simulink model "imageReceiveExample1"  (R2014a)
settings: Solver=FixedStepDiscrete  StartTime=0.0  StopTime=inf  RelTol=1e-3
undefined symbols (not defined in the file): gray, Rec, SDTV
libraries: dspmtrx3 x6, visionconversions x4, visionsinks x3, dspvision x2, ARdrone_video_lib x2
settings Model: xpc_rtwmakecfg_data=_jpeg_  Creator=Catarina  LastModifiedBy=Catarina

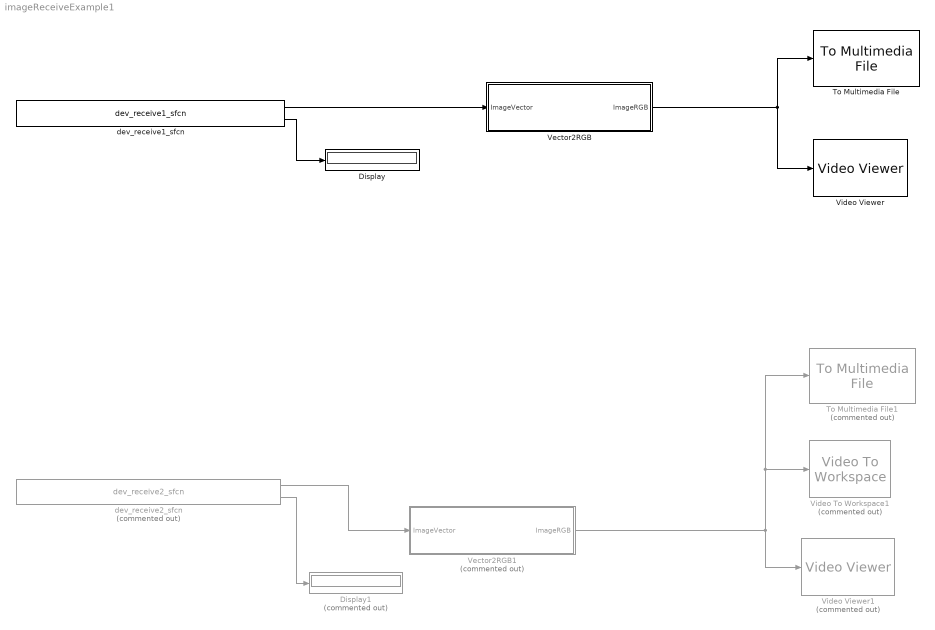
== system imageReceiveExample1 ==
  Display : Display
  Display1 : Display  Commented=on
  To Multimedia File : dspvision/To Multimedia File  outputFilename=output.avi  streamSelection=Video only  videoCompressor=None (uncompressed)  audioCompressor=None (uncompressed)  imagePorts=One multidimensional signal  fileType=AVI  audioDatatype=Determine from input data type  fourcc=RGB  videoQuality=75  mj2000CompFactor=10
  To Multimedia File1 : dspvision/To Multimedia File  Commented=on  outputFilename=output2.avi  streamSelection=Video only  videoCompressor=None (uncompressed)  audioCompressor=None (uncompressed)  imagePorts=One multidimensional signal  fileType=AVI  audioDatatype=Determine from input data type  fourcc=RGB  videoQuality=75  mj2000CompFactor=10
  Vector2RGB : Subsystem
  Vector2RGB1 : Subsystem  Commented=on
  Video To Workspace1 : visionsinks/Video To Workspace  Commented=on  VariableName=vout2  NumInputs=1  DataLimit=10  DecimationFactor=1  LogFi=off  InPortLabels=R|G|B
  Video Viewer : visionsinks/Video Viewer  inputType=Obsolete7b  imagePorts=One multidimensional signal  useColorMap=off  colormapValue=gray(256)  specRange=off  minInputVal=0  maxInputVal=255  FigPos=[1 1038 1920 938]  AxisZoom=on  trueSizedOnce=off  OpenAtMdlStart=on  DefaultConfigurationName=vipscopes.VideoViewerScopeCfg
  Video Viewer1 : visionsinks/Video Viewer  Commented=on  inputType=Obsolete7b  imagePorts=One multidimensional signal  useColorMap=off  colormapValue=gray(256)  specRange=off  minInputVal=0  maxInputVal=255  FigPos=[1 1038 1916 938]  AxisZoom=on  trueSizedOnce=off  OpenAtMdlStart=on  DefaultConfigurationName=vipscopes.VideoViewerScopeCfg
  dev_receive1_sfcn : ARdrone_video_lib/dev_receive1_sfcn  SFunctionSpec=double y2 = imageReceive1(uint8 y1[1843200], int32 work1[1])  SParameter1=[25500]  SampleTime=1/20  ShowSpec=on
  dev_receive2_sfcn : ARdrone_video_lib/dev_receive2_sfcn  Commented=on  SFunctionSpec=double y2 = imageReceive2(uint8 y1[153600], int32 work1[1])  SParameter1=ones([1 1 ])  SampleTime=-1  ShowSpec=on
  wires:
  Vector2RGB1/1(ImageRGB) -> Video Viewer1/1, To Multimedia File1/1, Video To Workspace1/1
  Vector2RGB/1(ImageRGB) -> Video Viewer/1, To Multimedia File/1
  dev_receive1_sfcn/1 -> Vector2RGB/1(ImageVector)
  dev_receive1_sfcn/2 -> Display/1
  dev_receive2_sfcn/1 -> Vector2RGB1/1(ImageVector)
  dev_receive2_sfcn/2 -> Display1/1

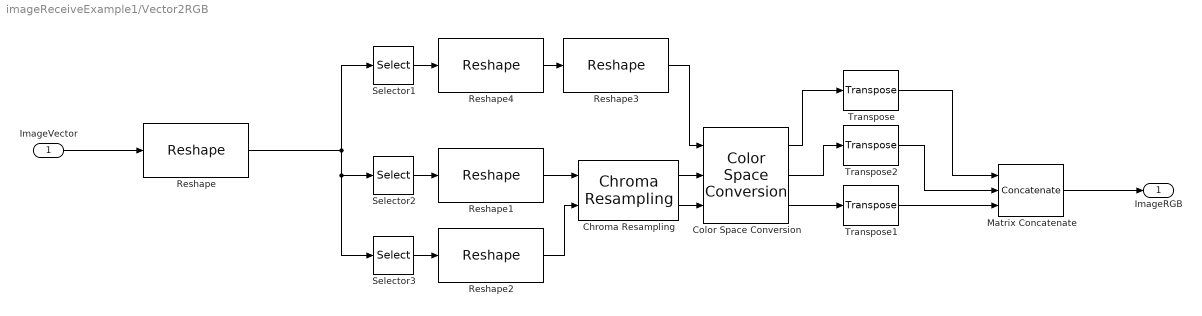
== system imageReceiveExample1/Vector2RGB ==
  ImageVector : Inport
  Chroma Resampling : visionconversions/Chroma Resampling  resampling=4:2:2 to 4:4:4  interpolation=pixel replication  antialiasing=Default  hcoeff=[0.2 0.6 0.2]  vcoeff=[0.5 0.5]  isInputTransposed=on
  Color Space Conversion : visionconversions/Color Space  Conversion  conversion=Obsolete  conversionActive=Y'CbCr to R'G'B'  wp_str=D65  rec=Rec. 601 (SDTV)  sys=1125/60/2:1  imagePorts=Separate color signals
  Matrix Concatenate : Concatenate  NumInputs=3  Mode=Multidimensional array  ConcatenateDimension=3
  Reshape : Reshape  OutputDimensionality=Customize  OutputDimensions=[4 1280*720*2/4]
  Reshape1 : Reshape  OutputDimensionality=Customize  OutputDimensions=[1280/2 720]
  Reshape2 : Reshape  OutputDimensionality=Customize  OutputDimensions=[1280/2 720]
  Reshape3 : Reshape  OutputDimensionality=Customize  OutputDimensions=[1280 720]
  Reshape4 : Reshape  OutputDimensionality=Customize  OutputDimensions=[4 1843200/8]
  Selector1 : Selector  NumberOfDimensions=2  InputPortWidth=3  IndexOptions=Index vector (dialog),Index vector (dialog)  Indices=[2 4],[1:460800]  OutputSizes=1,1
  Selector2 : Selector  NumberOfDimensions=2  InputPortWidth=3  IndexOptions=Index vector (dialog),Index vector (dialog)  Indices=1,[1:460800]  OutputSizes=1,1
  Selector3 : Selector  NumberOfDimensions=2  InputPortWidth=3  IndexOptions=Index vector (dialog),Index vector (dialog)  Indices=3,[1:460800]  OutputSizes=1,1
  Transpose : dspmtrx3/Transpose  Hermitian=off  overflowFlag=off
  Transpose1 : dspmtrx3/Transpose  Hermitian=off  overflowFlag=off
  Transpose2 : dspmtrx3/Transpose  Hermitian=off  overflowFlag=off
  ImageRGB : Outport
  wires:
  Transpose/1 -> Matrix Concatenate/1
  Selector2/1 -> Reshape1/1
  Selector3/1 -> Reshape2/1
  Color Space Conversion/3 -> Transpose1/1
  Selector1/1 -> Reshape4/1
  Reshape1/1 -> Chroma Resampling/1
  Color Space Conversion/1 -> Transpose/1
  Color Space Conversion/2 -> Transpose2/1
  Transpose1/1 -> Matrix Concatenate/3
  ImageVector/1 -> Reshape/1
  Reshape2/1 -> Chroma Resampling/2
  Chroma Resampling/2 -> Color Space Conversion/3
  Reshape3/1 -> Color Space Conversion/1
  Matrix Concatenate/1 -> ImageRGB/1
  Chroma Resampling/1 -> Color Space Conversion/2
  Reshape4/1 -> Reshape3/1
  Transpose2/1 -> Matrix Concatenate/2
  Reshape/1 -> Selector3/1, Selector2/1, Selector1/1

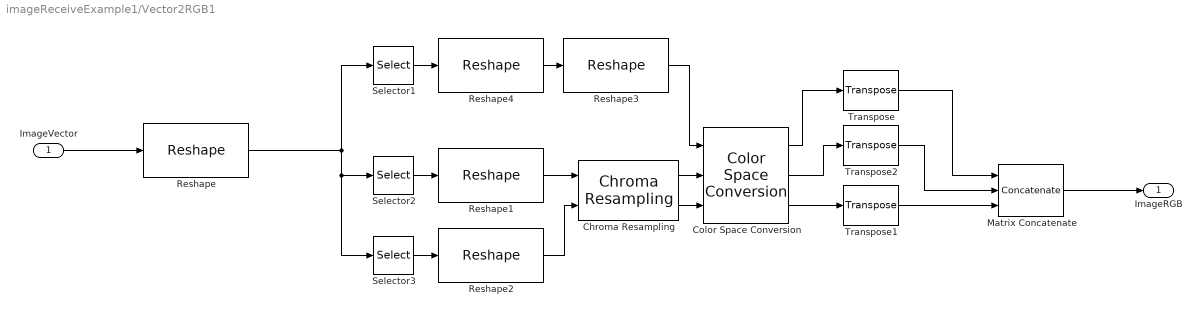
== system imageReceiveExample1/Vector2RGB1 ==
  ImageVector : Inport
  Chroma Resampling : visionconversions/Chroma Resampling  resampling=4:2:2 to 4:4:4  interpolation=pixel replication  antialiasing=Default  hcoeff=[0.2 0.6 0.2]  vcoeff=[0.5 0.5]  isInputTransposed=on
  Color Space Conversion : visionconversions/Color Space  Conversion  conversion=Obsolete  conversionActive=Y'CbCr to R'G'B'  wp_str=D65  rec=Rec. 601 (SDTV)  sys=1125/60/2:1  imagePorts=Separate color signals
  Matrix Concatenate : Concatenate  NumInputs=3  Mode=Multidimensional array  ConcatenateDimension=3
  Reshape : Reshape  OutputDimensionality=Customize  OutputDimensions=[4 320*240*2/4]
  Reshape1 : Reshape  OutputDimensionality=Customize  OutputDimensions=[320/2 240]
  Reshape2 : Reshape  OutputDimensionality=Customize  OutputDimensions=[320/2 240]
  Reshape3 : Reshape  OutputDimensionality=Customize  OutputDimensions=[320 240]
  Reshape4 : Reshape  OutputDimensionality=Customize  OutputDimensions=[4 38400/8]
  Selector1 : Selector  NumberOfDimensions=2  InputPortWidth=3  IndexOptions=Index vector (dialog),Index vector (dialog)  Indices=[2 4],[1:38400]  OutputSizes=1,1
  Selector2 : Selector  NumberOfDimensions=2  InputPortWidth=3  IndexOptions=Index vector (dialog),Index vector (dialog)  Indices=1,[1:38400]  OutputSizes=1,1
  Selector3 : Selector  NumberOfDimensions=2  InputPortWidth=3  IndexOptions=Index vector (dialog),Index vector (dialog)  Indices=3,[1:38400]  OutputSizes=1,1
  Transpose : dspmtrx3/Transpose  Hermitian=off  overflowFlag=off
  Transpose1 : dspmtrx3/Transpose  Hermitian=off  overflowFlag=off
  Transpose2 : dspmtrx3/Transpose  Hermitian=off  overflowFlag=off
  ImageRGB : Outport
  wires:
  Transpose/1 -> Matrix Concatenate/1
  Selector2/1 -> Reshape1/1
  Selector3/1 -> Reshape2/1
  Color Space Conversion/3 -> Transpose1/1
  Selector1/1 -> Reshape4/1
  Reshape1/1 -> Chroma Resampling/1
  Color Space Conversion/1 -> Transpose/1
  Color Space Conversion/2 -> Transpose2/1
  Transpose1/1 -> Matrix Concatenate/3
  ImageVector/1 -> Reshape/1
  Reshape2/1 -> Chroma Resampling/2
  Chroma Resampling/2 -> Color Space Conversion/3
  Reshape3/1 -> Color Space Conversion/1
  Matrix Concatenate/1 -> ImageRGB/1
  Chroma Resampling/1 -> Color Space Conversion/2
  Reshape4/1 -> Reshape3/1
  Transpose2/1 -> Matrix Concatenate/2
  Reshape/1 -> Selector3/1, Selector2/1, Selector1/1
